simulink model "WK_Maobi_writing25thDTP"  (Simulink 7.7)
settings: Solver=ode4  StartTime=0.0  StopTime=inf  FixedStep=sample_time  RelTol=1e-3
InitFcn:
  | sample_time=0.005;%0.004;%0.0025;%0.02;
  | DeltaT = 0.02;
  | g = 9.81;
  | H0 = g%0.3165;
  | Kl = 1;
  | 
  | Omega_r = 1.6;%for Horizontal reference
  | Zeta_r = 1; %for Horizontal reference
  | Omega = 1.8;%for Horizontal Control
  | Zeta = 0.5;    %for Horizontal Control
  | 
  | Omega_h_r = 2.5; %for vertical reference
  | Zeta_h_r = 1;  %for vertical reference
  | Omega_h = 2.7;    %for vertical control
  | Zeta_h = 0.8;         %for vertical control
  | PI=pi;
  | 
  | Mass = 1.15;
  | Acc_Max = 4;
  | Acc_Max_h = 4;
  | 
  | Max_RP = 60;
  | 
  | % for NN
  | n = 5;
  | r = 3;
  | n2 = 5;
  | NN_ST = 0.02;
  | 
  | GAMA_V = 6;
  | gama_V_e = 0.01;
  | 
  | GAMA_W = GAMA_V;
  | gama_W_e =0.01;
  | 
  | % deadzone
  | NN_Deadzone_Z = 0;
  | 
  | % inputs nomalizaton parameters
  | NN_Z_y_min = -3;
  | NN_Z_y_max = 0.5;
  | 
  | NN_Z_v_max = 8;
  | NN_Z_v_min = -NN_Z_v_max;
  | 
  | % alpha = 0.034;
  | alpha = 1;
  | % c_f = 0.0015;
  | c_f = 0.001;
  | c_y_tilt = 1*0.5;
  | 
  | %for WK paras
  | Heightcontrol = 0.08;
  | Scale_Factor=1;
  | yoffset=0;
  | 
  | load MaoBi_Oct04_2_int.mat
  | MB_Interp.time = [];
undefined symbols (not defined in the file or in its folder): DiscIntNeverNeededParam
libraries: simulink x7, dspadpt3 x3, X330_Control x2
(part 2 of 2)

== system WK_Maobi_writing25thDTP/Vicon_Data/Raw Quad Pose from Vicon/Process Vicon Raw Data1/Flip_pi1/Flip_0_to_2pi ==
  Angle : Inport
  Add : Sum
  Compare To Constant1 : simulink/Logic and Bit Operations/Compare To Constant  SystemSampleTime=-1  relop=<  const=0  LogicOutDataTypeMode=uint8  ZeroCross=off
  Constant : Constant  Value=2*pi
  Data Type Duplicate : DataTypeDuplicate
  Flip_2pi : Subsystem
      mask Type: Flip -2pi to 2pi
      mask Description: Flips the inputs into the range -2pi to +2pi
      mask Help: Flips the inputs into the range -2pi to +2pi
      mask Display: disp('Flip_2pi')
  Switch : Switch  Criteria=u2 ~= 0
  Angle_Flip : Outport
  wires:
  Flip_2pi/1(Angle_Flip) -> Compare To Constant1/1, Add/2, Switch/3
  Compare To Constant1/1 -> Switch/2
  Constant/1 -> Add/1
  Add/1 -> Switch/1
  Angle/1 -> Flip_2pi/1(Angle), Data Type Duplicate/2
  Switch/1 -> Angle_Flip/1, Data Type Duplicate/1

== system WK_Maobi_writing25thDTP/Vicon_Data/Raw Quad Pose from Vicon/Process Vicon Raw Data6/Flip_pi1/Flip_0_to_2pi ==
  Angle : Inport
  Add : Sum
  Compare To Constant1 : simulink/Logic and Bit Operations/Compare To Constant  SystemSampleTime=-1  relop=<  const=0  LogicOutDataTypeMode=uint8  ZeroCross=off
  Constant : Constant  Value=2*pi
  Data Type Duplicate : DataTypeDuplicate
  Flip_2pi : Subsystem
      mask Type: Flip -2pi to 2pi
      mask Description: Flips the inputs into the range -2pi to +2pi
      mask Help: Flips the inputs into the range -2pi to +2pi
      mask Display: disp('Flip_2pi')
  Switch : Switch  Criteria=u2 ~= 0
  Angle_Flip : Outport
  wires:
  Flip_2pi/1(Angle_Flip) -> Compare To Constant1/1, Add/2, Switch/3
  Compare To Constant1/1 -> Switch/2
  Constant/1 -> Add/1
  Add/1 -> Switch/1
  Angle/1 -> Flip_2pi/1(Angle), Data Type Duplicate/2
  Switch/1 -> Angle_Flip/1, Data Type Duplicate/1

== system WK_Maobi_writing25thDTP/Vicon_Data/Raw Quad Pose from Vicon/Process Vicon Raw Data7/Flip_pi1/Flip_0_to_2pi ==
  Angle : Inport
  Add : Sum
  Compare To Constant1 : simulink/Logic and Bit Operations/Compare To Constant  SystemSampleTime=-1  relop=<  const=0  LogicOutDataTypeMode=uint8  ZeroCross=off
  Constant : Constant  Value=2*pi
  Data Type Duplicate : DataTypeDuplicate
  Flip_2pi : Subsystem
      mask Type: Flip -2pi to 2pi
      mask Description: Flips the inputs into the range -2pi to +2pi
      mask Help: Flips the inputs into the range -2pi to +2pi
      mask Display: disp('Flip_2pi')
  Switch : Switch  Criteria=u2 ~= 0
  Angle_Flip : Outport
  wires:
  Switch/1 -> Data Type Duplicate/1, Angle_Flip/1
  Angle/1 -> Data Type Duplicate/2, Flip_2pi/1(Angle)
  Add/1 -> Switch/1
  Constant/1 -> Add/1
  Compare To Constant1/1 -> Switch/2
  Flip_2pi/1(Angle_Flip) -> Switch/3, Add/2, Compare To Constant1/1

== system WK_Maobi_writing25thDTP/Vicon_Data/Raw Quad Pose from Vicon/Process Vicon Raw Data1/Flip_pi1/Flip_0_to_2pi/Flip_2pi ==
  Angle : Inport
  Bias : Bias  Bias=-2*pi
  Constant : Constant  Value=2*pi
  Data Type Duplicate : DataTypeDuplicate
  Modulo : Math  Operator=mod  SaturateOnIntegerOverflow=on
  Sign1 : Signum
  Switch : Switch
  Angle_Flip : Outport
  wires:
  Angle/1 -> Modulo/1, Sign1/1, Data Type Duplicate/1
  Constant/1 -> Modulo/2
  Modulo/1 -> Bias/1, Switch/1
  Sign1/1 -> Switch/2
  Bias/1 -> Switch/3
  Switch/1 -> Angle_Flip/1, Data Type Duplicate/2

== system WK_Maobi_writing25thDTP/Vicon_Data/Raw Quad Pose from Vicon/Process Vicon Raw Data6/Flip_pi1/Flip_0_to_2pi/Flip_2pi ==
  Angle : Inport
  Bias : Bias  Bias=-2*pi
  Constant : Constant  Value=2*pi
  Data Type Duplicate : DataTypeDuplicate
  Modulo : Math  Operator=mod  SaturateOnIntegerOverflow=on
  Sign1 : Signum
  Switch : Switch
  Angle_Flip : Outport
  wires:
  Angle/1 -> Modulo/1, Sign1/1, Data Type Duplicate/1
  Constant/1 -> Modulo/2
  Modulo/1 -> Bias/1, Switch/1
  Sign1/1 -> Switch/2
  Bias/1 -> Switch/3
  Switch/1 -> Angle_Flip/1, Data Type Duplicate/2

== system WK_Maobi_writing25thDTP/Vicon_Data/Raw Quad Pose from Vicon/Process Vicon Raw Data7/Flip_pi1/Flip_0_to_2pi/Flip_2pi ==
  Angle : Inport
  Bias : Bias  Bias=-2*pi
  Constant : Constant  Value=2*pi
  Data Type Duplicate : DataTypeDuplicate
  Modulo : Math  Operator=mod  SaturateOnIntegerOverflow=on
  Sign1 : Signum
  Switch : Switch
  Angle_Flip : Outport
  wires:
  Switch/1 -> Data Type Duplicate/2, Angle_Flip/1
  Bias/1 -> Switch/3
  Sign1/1 -> Switch/2
  Modulo/1 -> Switch/1, Bias/1
  Constant/1 -> Modulo/2
  Angle/1 -> Data Type Duplicate/1, Sign1/1, Modulo/1

== matlab function Planning/Yaw Controller/MATLAB Function ==
  data: u input double; y output double
function y = fcn(u)
%#codegen
y = u;
if y > pi    
    y = y - 2*pi;
elseif y < -pi
        y = y + 2*pi;
end

== stateflow chart Planning/Trajectory Logic/UAV SF ==
  state Landing
    state Descending
      en:PosDesired = Pos;
      du:PosDesired[2] = (PerchPos[2]- PosDesired[2])*1*DeltaT + PosDesired[2] ;
    state CutThrottle
      du:HoverThrottle = (PerchPos[2] - HoverThrottle)*3*DeltaT + HoverThrottle ;
    (default) -> Descending
    Descending -> CutThrottle : [Pos[2] >(PerchPos[2] -0.1)]
  state Airborne
    state TakeOff
      du:HoverThrottle = (H0 - HoverThrottle)*3*DeltaT + HoverThrottle ;
    state Descent1
      descentrate=descentrate+0.02;
    state Descent
      en:PosDesired[2] = PerchPos[2]-0.50+descentrate;
    state Prelanding
      en:PosDesired[0] = PerchPos[0]; PosDesired[1] = PerchPos[1];PosDesired[2] = PerchPos[2]-0.8 ;
      descentrate=0;
    state SafyHover
      en:PosDesired = Pos; PosDesired[2]=-1.0;
    state D_Letter
      state drawing_straight_line2
        en:
        PosDesired[0]=-0.48, PosDesired[1]=-0.2,PosDesired[2]= -1.0;
        degree=4.712;
        height=0;
      state drawing_circle_line1
        en:
        PosDesired[0]=-0.48, PosDesired[1]=-0.2,PosDesired[2]= -1.0;
      state MBdown1
        en:
        PosDesired[0]=-0.48, PosDesired[1]=-0.2, PosDesired[2]=-0.55+height;
      state End_Point1
        en:
        PosDesired[0]=-0.48, PosDesired[1]=0.2,PosDesired[2]= -0.44;
      state MBup1
        en: PosDesired[2]= -1.0;
        height=0;
      state End_Point2
        en:
        PosDesired[0]=-0.48, PosDesired[1]=0.2,PosDesired[2]= -0.44;
      state drawing_circle_line2
        en:
        degree= degree+0.2617;
        PosDesired[2]=-0.44;
      state MBdown2
        en:
        PosDesired[0]=-0.48+0.2*cos(degree);
        PosDesired[1]=0.2*sin(degree);
        PosDesired[2]=-0.44;
      state MBup2
        en:
        PosDesired[2]= -1.0;
      state MBdown3
        en:
        PosDesired[0]=-0.48, PosDesired[1]=-0.2, PosDesired[2]=-0.55+height;
      state drawing_circle_line3
        en:
        height= height+0.01;
      state drawing_circle_line4
        en:
        height= height+0.01;
      drawing_straight_line2 -> MBdown1 : [(abs(PosDesired[0]-Pos[0])+abs(PosDesired[1]-Pos[1])) <0.02]
      Airborne.D_Letter.MBup1 -> Airborne.D_Letter.drawing_circle_line1 : [(abs(PosDesired[2]-Pos[2])) <0.02]
      Airborne.D_Letter.MBdown2 -> Airborne.D_Letter.drawing_circle_line2 [order 1] : [degree<7.853]
      MBdown1 -> Airborne.D_Letter.End_Point1 [order 2] : [PosDesired[2]>-0.44]
      Airborne.D_Letter.End_Point1 -> Airborne.D_Letter.MBup1 : [(abs(PosDesired[2]-Pos[2])) <0.02]
      Airborne.D_Letter.End_Point2 -> Airborne.D_Letter.MBup2 : [(abs(PosDesired[2]-Pos[2]))<0.02]
      Airborne.D_Letter.MBdown2 -> Airborne.D_Letter.End_Point2 [order 2] : [degree>7.853]
      Airborne.D_Letter.drawing_circle_line2 -> Airborne.D_Letter.MBdown2 : after (1,sec)
      Airborne.D_Letter.drawing_circle_line1 -> Airborne.D_Letter.MBdown3 : [(abs(PosDesired[0]-Pos[0]))+(abs(PosDesired[1]-Pos[1]))+(abs(PosDesired[2]-Pos[2])) <0.02]
      (default) -> drawing_straight_line2
      Airborne.D_Letter.MBdown3 -> Airborne.D_Letter.MBdown2 [order 2] : [PosDesired[2]>-0.44]
      MBdown1 -> Airborne.D_Letter.drawing_circle_line3 [order 1] : [PosDesired[2]<-0.44]
      Airborne.D_Letter.MBdown3 -> Airborne.D_Letter.drawing_circle_line4 [order 1] : [PosDesired[2]<-0.44]
      Airborne.D_Letter.drawing_circle_line3 -> MBdown1 : after (0.5,sec)
      Airborne.D_Letter.drawing_circle_line4 -> Airborne.D_Letter.MBdown3 : after (0.5,sec)
    state T_Letter
      state drawing_straight_line10
        en:
        PosDesired[0]=-0.35, PosDesired[1]=-0.2,PosDesired[2]= -1.0;
        height=0;
      state MBdown10
        en:
        PosDesired[0]=-0.35, PosDesired[1]=-0.2, PosDesired[2]=-0.55+height;
      state End_Point10
        en:
        PosDesired[0]=-0.15, PosDesired[1]=-0.2,PosDesired[2]= -0.44;
      state MBup10
        en: PosDesired[2]= -1.0; height=0;
      state drawing_straight_line11
        en:
        PosDesired[0]=-0.25, PosDesired[1]=-0.2,PosDesired[2]= -1.0;
      state MBdown11
        en:
        PosDesired[0]=-0.25, PosDesired[1]=-0.2, PosDesired[2]=-0.55+height;
      state Mid_Point10
        en:
        PosDesired[0]=-0.25, PosDesired[1]=0,PosDesired[2]= draw[2]-0.44;
      state End_Point11
        en:
        PosDesired[0]=-0.25, PosDesired[1]=0.2,PosDesired[2]= -0.44;
      state MBup11
        en:
        PosDesired[2]= -1.0;
      state MBdown12
        en:
        height=height+0.01
      state MBdown13
        en:
        height=height+0.01
      (default) -> drawing_straight_line10
      drawing_straight_line10 -> MBdown10 : [(abs(PosDesired[0]-Pos[0]))+(abs(PosDesired[1]-Pos[1])) <0.02]
      MBdown10 -> End_Point10 [order 2] : [PosDesired[2]>-0.44]
      End_Point10 -> MBup10 : [(abs(PosDesired[2]-Pos[2])) <0.02]
      MBup10 -> drawing_straight_line11 : [(abs(PosDesired[2]-Pos[2]))<0.01]
      drawing_straight_line11 -> MBdown11 : [(abs(PosDesired[0]-Pos[0]))+(abs(PosDesired[1]-Pos[1])) <0.02]
      MBdown11 -> Mid_Point10 [order 2] : [PosDesired[2]>-0.44]
      Mid_Point10 -> End_Point11 : after (1,sec)
      End_Point11 -> MBup11 : [(abs(PosDesired[2]-Pos[2]))<0.02]
      MBdown13 -> MBdown11 : after (0.5,sec)
      MBdown10 -> MBdown12 [order 1] : [PosDesired[2]<-0.44]
      MBdown11 -> MBdown13 [order 1] : [PosDesired[2]<-0.44]
      MBdown12 -> MBdown10 : after (0.5,sec)
    state P_Letter
      state drawing_straight_line20
        en:
        PosDesired[0]=-0.12, PosDesired[1]=-0.2,PosDesired[2]= -1.0;
        degree=4.712; height=0;
      state MBdown20
        en:
        height=height+0.01;
      state End_Point20
        en:
        PosDesired[0]=-0.12, PosDesired[1]=0.2,PosDesired[2]= -0.44;
      state MBup20
        en: PosDesired[2]= -1.0; height=0;
      state drawing_circle_line20
        en:
        PosDesired[0]=-0.12, PosDesired[1]=-0.2,PosDesired[2]= -1.0;
      state MBdown21
        en:
        PosDesired[0]=-0.12+0.1*cos(degree);
        PosDesired[1]=-0.1+0.1*sin(degree);
        PosDesired[2]=-0.44;
      state drawing_circle_line21
        en:
        degree= degree+0.2617;
        PosDesired[2]=-0.44;
      state End_Point21
        en:
        PosDesired[0]=-0.12, PosDesired[1]=0,PosDesired[2]= -0.44;
      state MBup21
        en:
        PosDesired[2]= -1.0;
        height=0;
      state MBdown22
        en:
        PosDesired[0]=-0.12, PosDesired[1]=-0.2, PosDesired[2]=-0.55+height;
      state MBdown23
        en:
        height=height+0.01;
      state drawing_circle_line22
        en:
        PosDesired[0]=-0.12, PosDesired[1]=-0.2,PosDesired[2]= -0.55+height;
      (default) -> drawing_straight_line20
      drawing_straight_line20 -> MBdown22 : [(abs(PosDesired[0]-Pos[0]))+(abs(PosDesired[1]-Pos[1])) <0.02]
      End_Point20 -> MBup20 : [(abs(PosDesired[2]-Pos[2])) <0.02]
      MBup20 -> drawing_circle_line20 : [abs(PosDesired[2]-Pos[2])<0.02]
      MBdown22 -> End_Point20 [order 2] : [PosDesired[2] >0.44]
      MBdown21 -> drawing_circle_line21 [order 1] : [degree<7.853]
      drawing_circle_line21 -> MBdown21 : after (1,sec)
      MBdown21 -> End_Point21 [order 2] : [degree>7.853]
      drawing_circle_line20 -> drawing_circle_line22 : [(abs(PosDesired[0]-Pos[0]))+(abs(PosDesired[1]-Pos[1]))+(abs(PosDesired[2]-Pos[2])) <0.02]
      End_Point21 -> MBup21 : [(abs(PosDesired[2]-Pos[2]))<0.02]
      MBdown23 -> drawing_circle_line22 : after(0.5,sec)
      drawing_circle_line22 -> MBdown21 [order 2] : [PosDesired[2]>-0.44]
      MBdown20 -> MBdown22 : after(0.5,sec)
      MBdown22 -> MBdown20 [order 1] : [PosDesired[2]<-0.44]
      drawing_circle_line22 -> MBdown23 [order 1] : [PosDesired[2]<-0.44]
    state A2_Letter
      state drawing_straight_line30
        en:
        PosDesired[0]=-0.545, PosDesired[1]=-0.1,PosDesired[2]= -1.0;
        degree=3.1415; height=0;
      state MBdown30
        en:
        PosDesired[0]=-0.545+0.1*cos(degree);
        PosDesired[1]=0.1+0.1*sin(degree);
        PosDesired[2]=-0.44;
      state drawing_circle_line30
        en:
        degree= degree+0.2617;
        PosDesired[2]=-0.44;
      state End_Point30
        en:
        PosDesired[0]=-0.345, PosDesired[1]=-0.1,PosDesired[2]= -0.44;
      state MBdown34
        en:
        PosDesired[0]=-0.545;
        PosDesired[1]=0.1;
        PosDesired[2]=-0.55+height;
      state drawing_circle_line31
        en:
        height=height+0.01;
      state MBdown31
        en:
        PosDesired[0]=-0.345, PosDesired[1]=-0.1, PosDesired[2]=-0.44;
      state drawing_diagonal_line_mid30
        en:
        PosDesired[0]=-0.445, PosDesired[1]=0.05,PosDesired[2]= -0.44;
      state drawing_diagonal_line_end30
        en:
        PosDesired[0]=-0.545, PosDesired[1]=0.2,PosDesired[2]=-0.44;
      state drawing_straight_line31
        en:
        PosDesired[0]=-0.545, PosDesired[1]=0.2,PosDesired[2]= -1.0; height=0;
      state MBdown33
        en:
        PosDesired[0]=-0.545, PosDesired[1]=0.2, PosDesired[2]=-0.55+height;
      state End_Point31
        en:
        PosDesired[0]=-0.345, PosDesired[1]=0.2,PosDesired[2]= -0.44;
      state MBup32
        en: PosDesired[2]= -1.0;height=0;
      state drawing_circle_line32
        en:
        height=height+0.01;
      (default) -> drawing_straight_line30
      drawing_straight_line30 -> MBdown34 : [(abs(PosDesired[0]-Pos[0]))+(abs(PosDesired[1]-Pos[1]))+(abs(PosDesired[2]-Pos[2])) <0.02]
      drawing_circle_line30 -> MBdown30 : after (1,sec)
      MBdown30 -> drawing_circle_line30 [order 1] : [degree<6.283]
      End_Point30 -> MBdown31 : [(abs(PosDesired[2]-Pos[2])) <0.02]
      MBdown30 -> End_Point30 [order 2] : [degree > 6.283]
      MBdown34 -> MBdown30 [order 2] : [PosDesired[2]>-0.44]
      MBdown31 -> drawing_diagonal_line_mid30 : [(PosDesired[2]-Pos[2])<0.02]
      drawing_diagonal_line_mid30 -> drawing_diagonal_line_end30 : after(1,sec)
      drawing_diagonal_line_end30 -> drawing_straight_line31 : [(abs(PosDesired[2]-Pos[2])) <0.02]
      drawing_circle_line31 -> MBdown34 : after (0.5,sec)
      drawing_straight_line31 -> MBdown33 : [(abs(PosDesired[0]-Pos[0]))+(abs(PosDesired[1]-Pos[1])) <0.02]
      MBdown33 -> End_Point31 [order 2] : [(abs(PosDesired[2]-Pos[2])) <0.02]
      End_Point31 -> MBup32 : [(abs(PosDesired[2]-Pos[2])) <0.02]
      MBdown34 -> drawing_circle_line31 [order 1] : [PosDesired[2]<-0.44]
      MBdown33 -> drawing_circle_line32 [order 1] : [PosDesired[2]<-0.44]
      drawing_circle_line32 -> MBdown33 : after (0.5,sec)
    state SafyHover1
      en:PosDesired = Pos; PosDesired[2]=-1.0;
    state A5_Letter1
      state drawing_straight_line100
        en:
        PosDesired[0]=-0.95, PosDesired[1]=-0.2,PosDesired[2]= -1.0;
        degree=4.712;
        height=0;
      state MBdown100
        en:
        PosDesired[0]=-0.95, PosDesired[1]=-0.2, PosDesired[2]=-0.55+height;
      state drawing_circle_line3
        en:
        height= height+0.01;
      state End_Point1
        en:
        PosDesired[0]=-0.295, PosDesired[1]=0.2,PosDesired[2]= -0.44;
      state MBup1
        en: PosDesired[2]= -1.0;
        height=0;
      state drawing_circle_line1
        en:
        PosDesired[0]=-0.48, PosDesired[1]=-0.2,PosDesired[2]= -1.0;
      state drawing_circle_line4
        en:
        height= height+0.01;
      state MBdown3
        en:
        PosDesired[0]=-0.48, PosDesired[1]=-0.2, PosDesired[2]=-0.55+height;
      state MBdown2
        en:
        PosDesired[0]=-0.48+0.2*cos(degree);
        PosDesired[1]=0.2*sin(degree);
        PosDesired[2]=-0.44;
      state drawing_circle_line2
        en:
        degree= degree+0.2617;
        PosDesired[2]=-0.44;
      state End_Point2
        en:
        PosDesired[0]=-0.48, PosDesired[1]=0.2,PosDesired[2]= -0.44;
      state MBup2
        en:
        PosDesired[2]= -1.0;
      (default) -> drawing_straight_line100
      drawing_straight_line100 -> MBdown100 : [(abs(PosDesired[0]-Pos[0])+abs(PosDesired[1]-Pos[1])) <0.02]
      MBdown100 -> Airborne.A5_Letter1.drawing_circle_line3 [order 1] : [PosDesired[2]<-0.44]
      Airborne.A5_Letter1.drawing_circle_line3 -> MBdown100 : after (0.5,sec)
      MBdown100 -> Airborne.A5_Letter1.End_Point1 [order 2] : [PosDesired[2]>-0.44]
      Airborne.A5_Letter1.End_Point1 -> Airborne.A5_Letter1.MBup1 : [(abs(PosDesired[2]-Pos[2])) <0.02]
      Airborne.A5_Letter1.MBup1 -> Airborne.A5_Letter1.drawing_circle_line1 : [(abs(PosDesired[2]-Pos[2])) <0.02]
      Airborne.A5_Letter1.drawing_circle_line1 -> Airborne.A5_Letter1.MBdown3 : [(abs(PosDesired[0]-Pos[0]))+(abs(PosDesired[1]-Pos[1]))+(abs(PosDesired[2]-Pos[2])) <0.02]
      Airborne.A5_Letter1.MBdown3 -> Airborne.A5_Letter1.drawing_circle_line4 [order 1] : [PosDesired[2]<-0.44]
      Airborne.A5_Letter1.drawing_circle_line4 -> Airborne.A5_Letter1.MBdown3 : after (0.5,sec)
      Airborne.A5_Letter1.MBdown3 -> Airborne.A5_Letter1.MBdown2 [order 2] : [PosDesired[2]>-0.44]
      Airborne.A5_Letter1.MBdown2 -> Airborne.A5_Letter1.drawing_circle_line2 [order 1] : [degree<7.853]
      Airborne.A5_Letter1.drawing_circle_line2 -> Airborne.A5_Letter1.MBdown2 : after (1,sec)
      Airborne.A5_Letter1.MBdown2 -> Airborne.A5_Letter1.End_Point2 [order 2] : [degree>7.853]
      Airborne.A5_Letter1.End_Point2 -> Airborne.A5_Letter1.MBup2 : [(abs(PosDesired[2]-Pos[2]))<0.02]
    Descent -> Prelanding [order 1] : after (5,sec)
    (default) -> TakeOff : {PosDesired = Pos;  PosDesired[2] =-1.2;}
    SafyHover -> Prelanding : after (3, sec)
    Descent1 -> Descent : after (0.5,sec)
    Prelanding -> Descent : [PerchError < 0.01]
    Descent -> Descent1 [order 2] : [PerchError < 0.02]
    TakeOff -> SafyHover [order 2] : [RC[5] > 0.5]
    D_Letter -> SafyHover1 : [RC[5] > 0.5]
    TakeOff -> A2_Letter [order 1] : after (5,sec)
    P_Letter -> SafyHover1 : [RC[5] > 0.5]
    Airborne.D_Letter.MBup2 -> T_Letter : [(abs(PosDesired[2]-Pos[2]))<0.02]
    MBup11 -> P_Letter : [(abs(PosDesired[2]-Pos[2]))<0.02]
    A2_Letter -> SafyHover1 : [RC[5] > 0.5]
    SafyHover1 -> Prelanding : after(3,sec)
    T_Letter -> SafyHover1 : [RC[5] > 0.5]
    MBup32 -> A5_Letter1 : [abs(PosDesired[2]-Pos[2])<0.02]
  (default) -> Landing : {HoverThrottle = 0;}
  Airborne -> Landing : [RC[6] < -0.5]
  Landing -> Airborne : [RC[6] > 0.5]
  data: PosDesired output double size=4; HoverThrottle output double size=1; Mode output uint8 size=1; RC input double size=8; Pos input double size=4; PerchPos input double size=4; DeltaT parameter double size=1; H0 parameter double size=1; Kl parameter double size=1; VelCmd local double size=2 =0; PWM output double; PerchError input double; PI parameter double size=1; draw input double size=3; descentrate local double; degree local double; height local double
